simulink model "chap8_1sim"  (R2015a)
settings: Solver=ode45  StartTime=0.0  StopTime=30  RelTol=1e-3
settings Model: Creator=zhr  LastModifiedBy=zhr

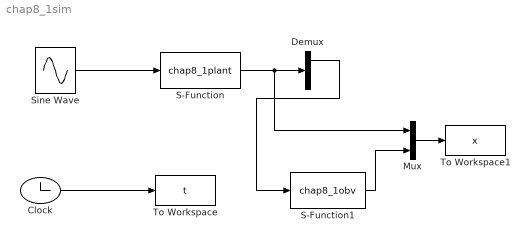
== system chap8_1sim ==
  Clock : Clock
  Demux : Demux  Outputs=2
  Mux : Mux  Inputs=2
  S-Function : S-Function  FunctionName=chap8_1plant
  S-Function1 : S-Function  FunctionName=chap8_1obv
  Sine Wave : Sin  SampleTime=0
  To Workspace : ToWorkspace  VariableName=t  SampleTime=-1
  To Workspace1 : ToWorkspace  VariableName=x  SampleTime=-1
  wires:
  Sine Wave/1 -> S-Function/1
  Clock/1 -> To Workspace/1
  S-Function/1 -> Mux/1, Demux/1
  Demux/1 -> S-Function1/1
  S-Function1/1 -> Mux/2
  Mux/1 -> To Workspace1/1
